simulink model "p1_e6"  (R2023b)
settings: Solver=FixedStepDiscrete  StartTime=0.0  StopTime=40  FixedStep=1  RelTol=1e-3
settings Model: LastModifiedBy=enrique

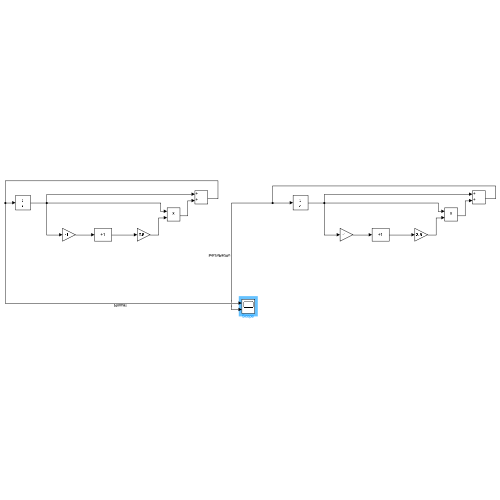
[thumbnail: Simulink's stored preview of the top-level diagram]
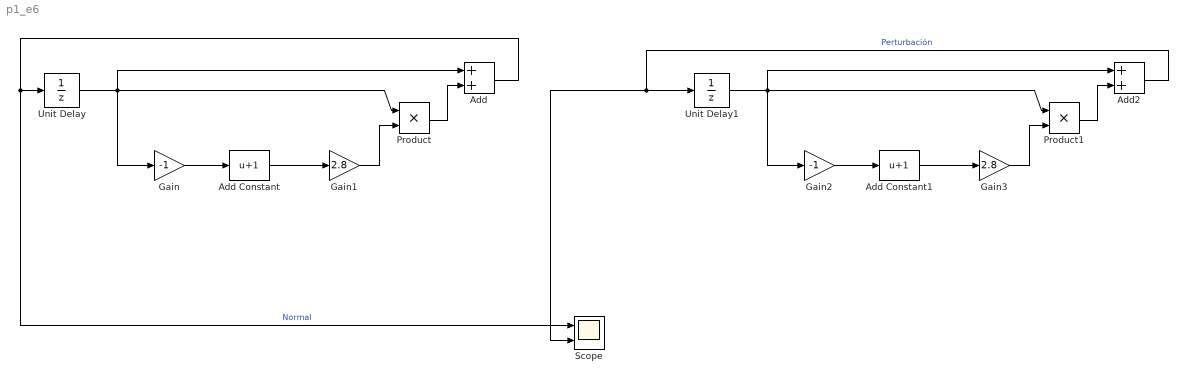
== system p1_e6 ==
  Add : Sum
  Add Constant : Bias  Bias=1  SaturateOnIntegerOverflow=off
  Add Constant1 : Bias  Bias=1  SaturateOnIntegerOverflow=off
  Add2 : Sum
  Gain : Gain  Gain=-1
  Gain1 : Gain  Gain=2.8
  Gain2 : Gain  Gain=-1
  Gain3 : Gain  Gain=2.8
  Product : Product
  Product1 : Product
  Scope : Scope  NumInputPorts=2
  Unit Delay : UnitDelay  InitialCondition=1.34  SampleTime=-1  HasFrameUpgradeWarning=on
  Unit Delay1 : UnitDelay  InitialCondition=1.34+(rand()*0.00001)  SampleTime=-1  HasFrameUpgradeWarning=on
  wires:
  Add Constant/1 -> Gain1/1
  Gain/1 -> Add Constant/1
  Unit Delay/1 -> Add/1, Gain/1, Product/1
  Gain1/1 -> Product/2
  Product/1 -> Add/2
  Add/1 -> Scope/1, Unit Delay/1  "Normal"
  Gain2/1 -> Add Constant1/1
  Product1/1 -> Add2/2
  Gain3/1 -> Product1/2
  Unit Delay1/1 -> Add2/1, Gain2/1, Product1/1
  Add Constant1/1 -> Gain3/1
  Add2/1 -> Scope/2, Unit Delay1/1  "Perturbación"
